simulink model "LAB1"  (Simulink 7.5)
settings: Solver=ode3  StartTime=0.0  StopTime=0.1  FixedStep=0.0001  RelTol=1e-3
settings Model: Creator=danbo324  LastModifiedBy=danbo324

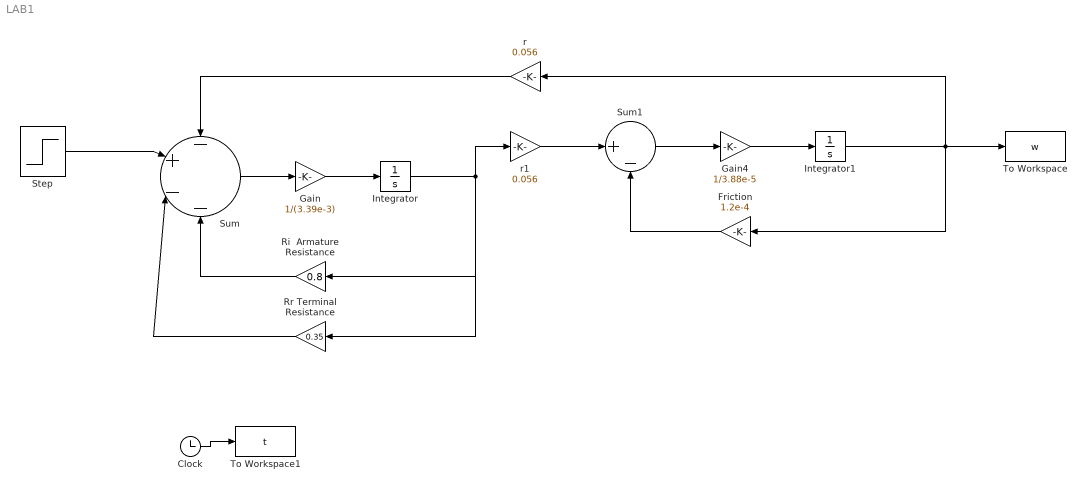
== system LAB1 ==
  Clock : Clock
      settings: Decimation=10
  Friction : Gain  Gain=1.2e-4  ParameterDataType=fixdt(1, 16)  ParameterScaling=2^0  OutDataType=fixdt(1, 16)  OutScaling=2^0
  Gain : Gain  Gain=1/(3.39e-3)  ParameterDataType=fixdt(1, 16)  ParameterScaling=2^0  OutDataType=fixdt(1, 16)  OutScaling=2^0
  Gain4 : Gain  Gain=1/3.88e-5  ParameterDataType=fixdt(1, 16)  ParameterScaling=2^0  OutDataType=fixdt(1, 16)  OutScaling=2^0
  Integrator : Integrator
  Integrator1 : Integrator
  Ri  Armature Resistance : Gain  Gain=0.8  ParameterDataType=fixdt(1, 16)  ParameterScaling=2^0  OutDataType=fixdt(1, 16)  OutScaling=2^0
  Rr Terminal Resistance : Gain  Gain=0.35  ParameterDataType=fixdt(1, 16)  ParameterScaling=2^0  OutDataType=fixdt(1, 16)  OutScaling=2^0
  Step : Step  Time=0  After=10  SampleTime=0
  Sum : Sum  Inputs=-+--  OutDataType=fixdt(1, 16)  OutScaling=2^0
  Sum1 : Sum  Inputs=|+-  OutDataType=fixdt(1, 16)  OutScaling=2^0
  To Workspace : ToWorkspace  VariableName=w  SampleTime=-1  SaveFormat=Array
  To Workspace1 : ToWorkspace  VariableName=t  SampleTime=-1  SaveFormat=Array
  r : Gain  Gain=0.056  ParameterDataType=fixdt(1, 16)  ParameterScaling=2^0  OutDataType=fixdt(1, 16)  OutScaling=2^0
  r1 : Gain  Gain=0.056  ParameterDataType=fixdt(1, 16)  ParameterScaling=2^0  OutDataType=fixdt(1, 16)  OutScaling=2^0
  wires:
  Gain/1 -> Integrator/1
  Integrator/1 -> Rr Terminal Resistance/1, r1/1, Ri  Armature Resistance/1
  Ri  Armature Resistance/1 -> Sum/4
  Rr Terminal Resistance/1 -> Sum/3
  Sum/1 -> Gain/1
  r1/1 -> Sum1/1
  Sum1/1 -> Gain4/1
  Gain4/1 -> Integrator1/1
  Integrator1/1 -> Friction/1, To Workspace/1, r/1
  Friction/1 -> Sum1/2
  r/1 -> Sum/1
  Step/1 -> Sum/2
  Clock/1 -> To Workspace1/1
